simulink model "s2"  (R2023b)
settings: Solver=ode45  StartTime=0  StopTime=1  RelTol=1e-3
settings Model: Creator=t3  LastModifiedBy=t3

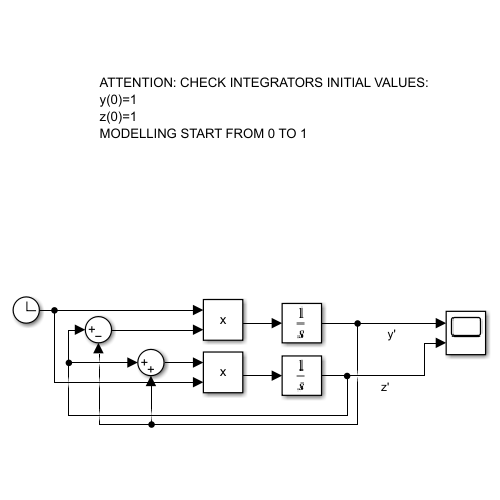
[thumbnail: Simulink's stored preview of the top-level diagram]
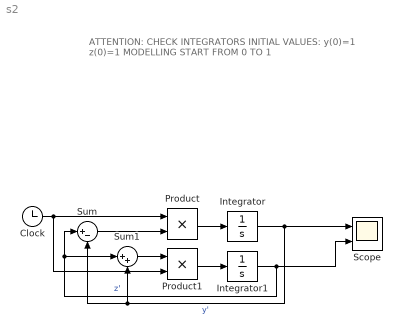
== system s2 ==
  note: ATTENTION: CHECK INTEGRATORS INITIAL VALUES:
      | y(0)=1
      | z(0)=1
      | MODELLING START FROM 0 TO 1
  Clock : Clock
  Integrator : Integrator  InitialCondition=1
  Integrator1 : Integrator  InitialCondition=1
  Product : Product
  Product1 : Product
  Scope : Scope  NumInputPorts=2
  Sum : Sum  Inputs=|+-
  Sum1 : Sum  Inputs=|++
  wires:
  Integrator/1 -> Sum1/2, Sum/2, Scope/1  "y'"
  Integrator1/1 -> Sum1/1, Sum/1, Scope/2  "z'"
  Product/1 -> Integrator/1
  Product1/1 -> Integrator1/1
  Clock/1 -> Product1/2, Product/1
  Sum/1 -> Product/2
  Sum1/1 -> Product1/1
